simulink model "hcu_main_ADASwEPS"  (Simulink 8.2)
settings: Solver=FixedStepDiscrete  StartTime=0.0  StopTime=inf  FixedStep=0.001  RelTol=1e-3
PostLoadFcn:
  | , if any(exist('dsrtsu_mdlpostloadfcn', 'file') == [2, 3, 6]), try dsrtsu_mdlpostloadfcn('Execute', bdroot); catch fprintf('Error in PostLoadFcn (dsrtsu_mdlpostloadfcn) for model "%s":\n %s\n', bdroot, lasterr); end, end,
values from neighbouring files (symbols this model uses):
  C_TASK_1MS_S = (	C_TICK_TIME_S       )    [hcu_local_hdr.m]    (also in temp_ovrd_values.m = double(	0.001                  ))
  C_TICK_TIME_S = single(	0.005	    	)    [hcu_local_hdr.m]
  ENUM_EPSLFCSTATUS_ACTIVE = uint8(  2  )    [hcu_local_hdr.m]
  ENUM_EPSLFCSTATUS_TRANSITION = uint8(  3  )    [hcu_local_hdr.m]
  ENUM_EPSLKASTATUS_ACTIVE = uint8(  2  )    [hcu_local_hdr.m]
  ENUM_EPSMODEREQ_ANGLE = uint8(  1  )    [hcu_local_hdr.m]
  ENUM_EPSMODEREQ_INTERNAL = uint8(  0  )    [hcu_local_hdr.m]
  ENUM_EPSMODEREQ_TORQUE = uint8(  2  )    [hcu_local_hdr.m]
  ENUM_GEARPOSN_1ST = uint8(  1  )    [hcu_local_hdr.m]
  ENUM_GEARPOSN_2ND = uint8(  2  )    [hcu_local_hdr.m]
  ENUM_GEARPOSN_3RD = uint8(  3  )    [hcu_local_hdr.m]
  ENUM_GEARPOSN_4TH = uint8(  4  )    [hcu_local_hdr.m]
  ENUM_GEARPOSN_5TH = uint8(  5  )    [hcu_local_hdr.m]
  ENUM_GEARPOSN_6TH = uint8(  6  )    [hcu_local_hdr.m]
  ENUM_GEARPOSN_R = uint8(  7  )    [hcu_local_hdr.m]
  FALSE = boolean( 0 )    [hcu_local_hdr.m]
  TRUE = boolean( 1 )    [hcu_local_hdr.m]
undefined symbols (not defined in the file or in its folder): AISP_EPSCurrent_pct, AISP_TqASensorDelta_pct, AISP_TqBSensorDelta_pct, dHAL_IN, hal, INVALID_ABS1_TIMEOUT, INVALID_ABS2_TIMEOUT, INVALID_ABS3_TIMEOUT, INVALID_ABS4_TIMEOUT, INVALID_AC1_TIMEOUT, INVALID_ADASTORQ_REQ, INVALID_BCM1_TIMEOUT, INVALID_BCM2_TIMEOUT, INVALID_BOOSTER_VAC, INVALID_CSW1_TIMEOUT, INVALID_CUR_VEHDECE, INVALID_CURBRAKEDECE_REQ, INVALID_CURSTEERANG_REQ, INVALID_CURSTEERTQ_REQ, INVALID_ECM1_TIMEOUT, INVALID_ECM2_TIMEOUT, INVALID_ECM3_TIMEOUT, INVALID_ECM9_TIMEOUT, INVALID_ENG_TORQUE_FRICTIONAL, INVALID_ENG_TORQUE_INDICATED, INVALID_ENG_TORQUE_INDICATEDCOR, INVALID_ENG_TQ_MAX, INVALID_ENG_TQ_MIN, INVALID_EPAS2_TIMEOUT, INVALID_EPAS3_TIMEOUT, INVALID_EPB1_TIMEOUT, INVALID_EPS_BATTVOLT, INVALID_ESC_BATTVOLT, INVALID_GRADE, INVALID_HCU3_TIMEOUT, INVALID_HCU4_TIMEOUT, INVALID_HMI1_TIMEOUT, INVALID_HMI2_TIMEOUT, INVALID_LAT_ACC, INVALID_LONG_ACC, INVALID_MC_PRESSURE, INVALID_METER1_TIMEOUT, INVALID_METER3_TIMEOUT, INVALID_METER_VEHSPD, INVALID_ODO_METER, INVALID_OUTSIDE_TEMP, INVALID_PARKBRAKEBIND_STAT, INVALID_PEDALTQ_REQ, INVALID_SAS1_TIMEOUT, INVALID_SAS_ANGLE, INVALID_SHIFTER_POSN, INVALID_TCM1_TIMEOUT, INVALID_TCM2_TIMEOUT, INVALID_VCU1_TIMEOUT, INVALID_VCU2_TIMEOUT, INVALID_VEH_CRASH, INVALID_VEH_SPD, INVALID_WHEEL_SPD, INVALID_YAW_RATE, KHAL_MssgIdObj1_num ... (+8)
libraries: simulink x147, hcu_lib x38, rti1401lib_dio_type3 x4, rtimmsu_dsrtlib x3, app x1, rtiethernetudplib x1, rti1401lib_adc_type4 x1, rti1401lib_dac_type3 x1, inp x1, lidr x1, outp x1
(part 11 of 15)

== system hcu_main_ADASwEPS/EPSS/EPSS/LFCStatusArbitration ==
  VISP_EPSModeReq_enum : Inport
  VEPSS_LFCContStatusAng_enum : Inport  Port=2
  VEPSS_LFCContStatusTq_enum : Inport  Port=3
  VEPSS_EPSLKAAbReason_enum : Inport  Port=4
  VEPSS_EPSLFCAbReasonAng_enum : Inport  Port=5
  VEPSS_EPSLFCAbReasonTq_enum : Inport  Port=6
  Constant1 : Constant  Value=ENUM_EPSMODEREQ_INTERNAL
  Constant6 : Constant  Value=ENUM_EPSMODEREQ_ANGLE
  Relational Operator1 : RelationalOperator  Operator===  OutDataTypeStr=boolean
  Relational Operator3 : RelationalOperator  Operator===  OutDataTypeStr=boolean
  Switch1 : Switch  Criteria=u2 ~= 0
  Switch2 : Switch  Criteria=u2 ~= 0
  Switch3 : Switch  Criteria=u2 ~= 0
  VEPSS_LFCContStatus_enum : Outport
  VEPSS_EPSADASAbReason_enum : Outport  Port=2
  wires:
  VISP_EPSModeReq_enum/1 -> Relational Operator1/1, Relational Operator3/1
  Constant6/1 -> Relational Operator3/2
  Relational Operator3/1 -> Switch2/2, Switch1/2
  VEPSS_LFCContStatusAng_enum/1 -> Switch1/1
  VEPSS_LFCContStatusTq_enum/1 -> Switch1/3
  Switch1/1 -> VEPSS_LFCContStatus_enum/1
  VEPSS_EPSLFCAbReasonAng_enum/1 -> Switch2/1
  VEPSS_EPSLFCAbReasonTq_enum/1 -> Switch2/3
  Constant1/1 -> Relational Operator1/2
  Switch2/1 -> Switch3/3
  VEPSS_EPSLKAAbReason_enum/1 -> Switch3/1
  Switch3/1 -> VEPSS_EPSADASAbReason_enum/1
  Relational Operator1/1 -> Switch3/2

== system hcu_main_ADASwEPS/EPSS/EPSS/PWM Output Limit ==
  VEPSS_SteerPWM_pct : Inport
  VISP_StrAng_deg : Inport  Port=2
  VISP_StrAngValid_flg : Inport  Port=3
  Data Type Conversion : DataTypeConversion
  KEPSS_LockLimitationDefault_rat : Constant  SampleTime=-1
  KEPSS_MotorDutyMaxLim_pct : Constant  Value=100  SampleTime=-1
  KEPSS_MotorDutyMinLim_pct : Constant  Value=-100  SampleTime=-1
  Limit : hcu_lib/Limit  SystemSampleTime=-1
  MEPSS_LockLimitation_rat : Lookup  InputValues=[-600 -540 0 540 600]  Table=[0.5 1 1 1 0.5]  LookUpMeth=Interpolation-Use End Values
      settings: AttributesFormatString="Input=\"%<InputValues>\"\\nOutput=\"%<Table>\""
  Product : Product
  Switch : Switch  Criteria=u2 ~= 0
  VEPSS_MotorDuty_pct_over : hcu_lib/Signal_over  parent_name=VEPSS_MotorDuty_pct  cal=0
  VEPSS_MotorDuty_pct : Outport
  wires:
  VEPSS_SteerPWM_pct/1 -> Limit/1
  VEPSS_MotorDuty_pct_over/1 -> Data Type Conversion/1
  KEPSS_MotorDutyMaxLim_pct/1 -> Limit/2
  KEPSS_MotorDutyMinLim_pct/1 -> Limit/3
  Data Type Conversion/1 -> VEPSS_MotorDuty_pct/1  "VEPSS_MotorDuty_pct"
  VISP_StrAng_deg/1 -> MEPSS_LockLimitation_rat/1
  MEPSS_LockLimitation_rat/1 -> Switch/1
  VISP_StrAngValid_flg/1 -> Switch/2
  KEPSS_LockLimitationDefault_rat/1 -> Switch/3
  Limit/1 -> Product/1
  Product/1 -> VEPSS_MotorDuty_pct_over/1
  Switch/1 -> Product/2  "VEPSS_LockLimitation_rat"

== system hcu_main_ADASwEPS/EPSS/EPSS/ShaftTorqueProcessor ==
  VISP_EPSTqOnShaft_Nm : Inport
  AddLPF : Constant  Value=0
  Data Type Conversion : DataTypeConversion
  LowPassFilter_50ms : DiscreteTransferFcn  Numerator=[0 0.019801326693245]  Denominator=[1 -0.980198673306755]
  NotchFilter1 : DiscreteTransferFcn  Numerator=[1 -1.994058244407765 0.995032825431470]  Denominator=[1 -1.974205875760737 0.975180456784442]
  NotchFilter2 : DiscreteTransferFcn  Numerator=[1 -1.991175781675417 0.993076280925535]  Denominator=[1 -1.963525487771149 0.965425987021267]
  NotchFilter3 : DiscreteTransferFcn  Numerator=[1 -1.986359097364601 0.990196128638903]  Denominator=[1 -1.941183460066831 0.945020491341134]
  NotchFilter4 : DiscreteTransferFcn  Numerator=[1 -1.978872423909787 0.986339393241381]  Denominator=[1 -1.924580367084394 0.932047336415988]
  NotchFilter5 : DiscreteTransferFcn  Numerator=[1 -1.956033818662219 0.973851168649108]  Denominator=[1 -1.853080945250230 0.870898295237120]
  Switch : Switch  Criteria=u2 ~= 0
  VEPSS_EPSTqOnShaftRaw_Nm : Outport
  VEPSS_EPSTqOnShaftFlt_Nm : Outport  Port=2
  wires:
  VISP_EPSTqOnShaft_Nm/1 -> Data Type Conversion/1, NotchFilter1/1
  NotchFilter1/1 -> NotchFilter2/1
  NotchFilter2/1 -> NotchFilter3/1
  NotchFilter3/1 -> NotchFilter4/1
  NotchFilter4/1 -> NotchFilter5/1
  NotchFilter5/1 -> LowPassFilter_50ms/1, Switch/3
  Data Type Conversion/1 -> VEPSS_EPSTqOnShaftRaw_Nm/1  "VEPSS_EPSTqOnShaftRaw_Nm"
  Switch/1 -> VEPSS_EPSTqOnShaftFlt_Nm/1  "VEPSS_EPSTqOnShaftFlt_Nm"
  LowPassFilter_50ms/1 -> Switch/1
  AddLPF/1 -> Switch/2

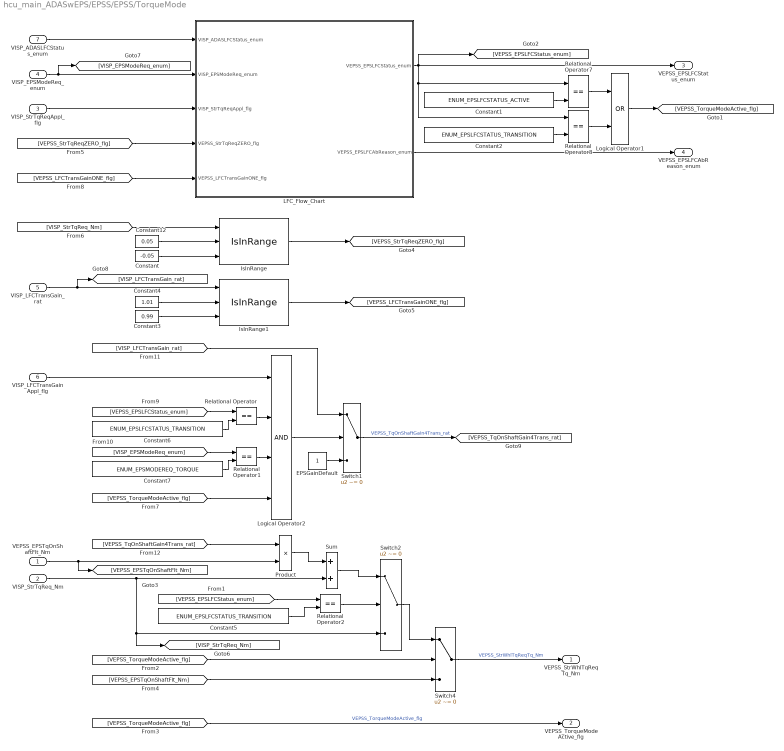
== system hcu_main_ADASwEPS/EPSS/EPSS/TorqueMode ==
  VEPSS_EPSTqOnShaftFlt_Nm : Inport
  VISP_StrTqReq_Nm : Inport  Port=2
  VISP_StrTqReqAppl_flg : Inport  Port=3
  VISP_EPSModeReq_enum : Inport  Port=4
  VISP_LFCTransGain_rat : Inport  Port=5
  VISP_LFCTransGainAppl_flg : Inport  Port=6
  VISP_ADASLFCStatus_enum : Inport  Port=7
  Constant : Constant  Value=-0.05
  Constant1 : Constant  Value=ENUM_EPSLFCSTATUS_ACTIVE
  Constant12 : Constant  Value=0.05
  Constant2 : Constant  Value=ENUM_EPSLFCSTATUS_TRANSITION
  Constant3 : Constant  Value=0.99
  Constant4 : Constant  Value=1.01
  Constant5 : Constant  Value=ENUM_EPSLFCSTATUS_TRANSITION
  Constant6 : Constant  Value=ENUM_EPSLFCSTATUS_TRANSITION
  Constant7 : Constant  Value=ENUM_EPSMODEREQ_TORQUE
  EPSGainDefault : Constant
  IsInRange : hcu_lib/IsInRange  SystemSampleTime=-1
  IsInRange1 : hcu_lib/IsInRange  SystemSampleTime=-1
  LFC_Flow_Chart : Stateflow chart  TreatAsAtomicUnit=on
  Logical Operator1 : Logic  Operator=OR  AllPortsSameDT=off  OutDataTypeStr=boolean
  Logical Operator2 : Logic  Inputs=4  AllPortsSameDT=off  OutDataTypeStr=boolean
  Product : Product
  Relational Operator{,1..2,7..8} (5 alike) : RelationalOperator  Operator===  OutDataTypeStr=boolean
  Sum : Sum
  Switch1 : Switch  Criteria=u2 ~= 0
  Switch2 : Switch  Criteria=u2 ~= 0
  Switch4 : Switch  Criteria=u2 ~= 0
  VEPSS_StrWhlTqReqTq_Nm : Outport
  VEPSS_TorqueModeActive_flg : Outport  Port=2
  VEPSS_EPSLFCStatus_enum : Outport  Port=3
  VEPSS_EPSLFCAbReason_enum : Outport  Port=4
  wires:
  Sum/1 -> Switch2/1
  VISP_StrTqReq_Nm/1 -> [VISP_StrTqReq_Nm], Switch2/3, Sum/2
  Switch4/1 -> VEPSS_StrWhlTqReqTq_Nm/1  "VEPSS_StrWhlTqReqTq_Nm"
  VEPSS_EPSTqOnShaftFlt_Nm/1 -> [VEPSS_EPSTqOnShaftFlt_Nm], Product/2
  Switch2/1 -> Switch4/1
  [VEPSS_TorqueModeActive_flg] -> Switch4/2
  [VEPSS_EPSLFCStatus_enum] -> Relational Operator2/1
  Constant5/1 -> Relational Operator2/2
  Relational Operator2/1 -> Switch2/2
  [VEPSS_EPSTqOnShaftFlt_Nm] -> Switch4/3
  [VEPSS_TorqueModeActive_flg] -> VEPSS_TorqueModeActive_flg/1  "VEPSS_TorqueModeActive_flg"
  [VISP_StrTqReq_Nm] -> IsInRange/1
  IsInRange/1 -> [VEPSS_StrTqReqZERO_flg]
  Constant/1 -> IsInRange/3
  Constant12/1 -> IsInRange/2
  LFC_Flow_Chart/1(VEPSS_EPSLFCStatus_enum) -> [VEPSS_EPSLFCStatus_enum], VEPSS_EPSLFCStatus_enum/1, Relational Operator8/1, Relational Operator7/1
  Constant1/1 -> Relational Operator7/2
  Constant2/1 -> Relational Operator8/2
  LFC_Flow_Chart/2(VEPSS_EPSLFCAbReason_enum) -> VEPSS_EPSLFCAbReason_enum/1
  Relational Operator8/1 -> Logical Operator1/2
  Relational Operator7/1 -> Logical Operator1/1
  Logical Operator1/1 -> [VEPSS_TorqueModeActive_flg]
  VISP_ADASLFCStatus_enum/1 -> LFC_Flow_Chart/1(VISP_ADASLFCStatus_enum)
  VISP_EPSModeReq_enum/1 -> [VISP_EPSModeReq_enum], LFC_Flow_Chart/2(VISP_EPSModeReq_enum)
  VISP_StrTqReqAppl_flg/1 -> LFC_Flow_Chart/3(VISP_StrTqReqAppl_flg)
  [VEPSS_StrTqReqZERO_flg] -> LFC_Flow_Chart/4(VEPSS_StrTqReqZERO_flg)
  VISP_LFCTransGain_rat/1 -> [VISP_LFCTransGain_rat], IsInRange1/1
  IsInRange1/1 -> [VEPSS_LFCTransGainONE_flg]
  Constant3/1 -> IsInRange1/3
  Constant4/1 -> IsInRange1/2
  [VEPSS_LFCTransGainONE_flg] -> LFC_Flow_Chart/5(VEPSS_LFCTransGainONE_flg)
  [VEPSS_EPSLFCStatus_enum] -> Relational Operator/1
  Constant6/1 -> Relational Operator/2
  VISP_LFCTransGainAppl_flg/1 -> Logical Operator2/1
  Relational Operator/1 -> Logical Operator2/2
  [VEPSS_TorqueModeActive_flg] -> Logical Operator2/4
  Logical Operator2/1 -> Switch1/2
  Switch1/1 -> [VEPSS_TqOnShaftGain4Trans_rat]  "VEPSS_TqOnShaftGain4Trans_rat"
  EPSGainDefault/1 -> Switch1/3
  [VISP_EPSModeReq_enum] -> Relational Operator1/1
  Constant7/1 -> Relational Operator1/2
  Relational Operator1/1 -> Logical Operator2/3
  [VISP_LFCTransGain_rat] -> Switch1/1
  Product/1 -> Sum/1
  [VEPSS_TqOnShaftGain4Trans_rat] -> Product/1

== system hcu_main_ADASwEPS/EPSS/model_info/EmptySubsystem ==

== system hcu_main_ADASwEPS/ISP/AngleProcessing/Timer ==
  Enable : EnablePort  StatesWhenEnabling=reset
  C_TASK_1MS_S : Constant  Value=C_TASK_1MS_S
  Sum : Sum  Inputs=|++
  Unit Delay : UnitDelay  SampleTime=-1
  Unit Delay1 : UnitDelay  SampleTime=-1
  Time_s : Outport  OutputWhenDisabled=reset  InitialOutput=[0]
  wires:
  C_TASK_1MS_S/1 -> Unit Delay1/1
  Sum/1 -> Unit Delay/1, Time_s/1  "Time_s"
  Unit Delay/1 -> Sum/2
  Unit Delay1/1 -> Sum/1

== system hcu_main_ADASwEPS/ISP/AngleProcessing/Triggered Absolute Angle Zero ==
  In : Inport
  Trigger : TriggerPort
  SteerAngValid_flg : Constant  Value=TRUE
  Out1 : Outport
  Out2 : Outport  Port=2
  wires:
  In/1 -> Out1/1
  SteerAngValid_flg/1 -> Out2/1

== system hcu_main_ADASwEPS/ISP/PassThrough/EPSDegTest ==
  PassThrough : Inport
  AmplitudeDeg_pct : Constant  Value=5
  Compare To Constant : simulink/Logic and Bit Operations/Compare To Constant  relop===  const=3.0  OutDataTypeStr=boolean
  Constant : Constant  Value=2*pi  OutDataTypeStr=single
  DegSetPt : Constant
  FrequencyDeg_Hz : Constant
  Multiport Switch1 : MultiPortSwitch  Inputs=4
  Product : Product  Inputs=3  RndMeth=Zero
  Product1 : Product  RndMeth=Zero
  TestModeDeg_Sw : Constant
  Timer : Subsystem
  Trigonometric Funcon : Trigonometry
  DegOut : Outport
  wires:
  Multiport Switch1/1 -> DegOut/1  "DegOut"
  PassThrough/1 -> Multiport Switch1/2
  DegSetPt/1 -> Multiport Switch1/3
  Product1/1 -> Multiport Switch1/4
  FrequencyDeg_Hz/1 -> Product/2
  Product/1 -> Trigonometric Funcon/1
  AmplitudeDeg_pct/1 -> Product1/2
  Trigonometric Funcon/1 -> Product1/1
  Constant/1 -> Product/3
  Timer/1(SineTime_s) -> Product/1
  TestModeDeg_Sw/1 -> Compare To Constant/1, Multiport Switch1/1
  Compare To Constant/1 -> Timer/Enable

== system hcu_main_ADASwEPS/ISP/TqProcessing/LowPassFilter ==
  Raw : Inport
  Constant1 : Constant  OutDataTypeStr=single  SampleTime=-1
  LowPassCoef : Constant  SampleTime=-1
  Product : Product  RndMeth=Zero
  Product1 : Product  RndMeth=Zero
  Sum1 : Sum  Inputs=+-
  Sum2 : Sum
  Unit Delay1 : UnitDelay  SampleTime=-1
  Out : Outport
  wires:
  Raw/1 -> Product/2
  Constant1/1 -> Sum1/1
  LowPassCoef/1 -> [LowPassCoef], Product/1
  [LowPassCoef] -> Sum1/2
  Unit Delay1/1 -> Product1/1
  Sum1/1 -> Product1/2
  Product/1 -> Sum2/1
  Product1/1 -> Sum2/2
  Sum2/1 -> Unit Delay1/1, Out/1

== system hcu_main_ADASwEPS/ISP/TqProcessing/TorqueValid ==
  TqA : Inport
  TqB : Inport  Port=2
  Abs1 : Abs
  FALSE : Constant  Value=FALSE  OutDataTypeStr=single  SampleTime=-1
  Relational Operator1 : RelationalOperator  Operator=<=  OutDataTypeStr=boolean
  Sum1 : Sum  Inputs=+-
  Switch1 : Switch  Criteria=u2 ~= 0
  TRUE : Constant  Value=TRUE  OutDataTypeStr=single  SampleTime=-1
  TqValidThres_Nm : Constant  OutDataTypeStr=single  SampleTime=-1
  TqValid_flg : Outport
  wires:
  TRUE/1 -> Switch1/1
  TqValidThres_Nm/1 -> Relational Operator1/2
  Relational Operator1/1 -> Switch1/2
  Sum1/1 -> Abs1/1
  Abs1/1 -> Relational Operator1/1
  FALSE/1 -> Switch1/3
  Switch1/1 -> TqValid_flg/1  "TqValid_flg"
  TqA/1 -> Sum1/1
  TqB/1 -> Sum1/2

== system hcu_main_ADASwEPS/ISP/TqProcessing/TqSensorAZero ==
  VHAL_TqSensorADuty_pct : Inport
  TqSensorFlac_pct : Inport  Port=2
  KISP_EPSZeroReset_flg : Inport  Port=3
  Constant1 : Constant  Value=60  OutDataTypeStr=single  SampleTime=-1
  Constant2 : Constant  Value=50  OutDataTypeStr=single  SampleTime=-1
  Delay : Delay  DelayLength=1  InitialCondition=0
  Delay1 : Delay  DelayLength=1  InitialCondition=1
  Delay2 : Delay  DelayLength=1  InitialCondition=1
  FALSE : Constant  Value=FALSE
  Gain : Gain  Gain=-1
  IsInRange : hcu_lib/IsInRange  SystemSampleTime=-1
  IsInRange1 : hcu_lib/IsInRange  SystemSampleTime=-1
  KISP_CheckZeroTime_s : Constant  Value=3
  Latch : Subsystem
  Logical Operator : Logic  Operator=NOT  AllPortsSameDT=off  OutDataTypeStr=boolean
  Logical Operator1 : Logic  Operator=OR  AllPortsSameDT=off  OutDataTypeStr=boolean
  Logical Operator4 : Logic  AllPortsSameDT=off  OutDataTypeStr=boolean
  Relational Operator : RelationalOperator  Operator=<=  OutDataTypeStr=boolean
  Subtract : Sum  Inputs=+-
  Subtract1 : Sum  Inputs=+-
  Switch : Switch  Criteria=u2 ~= 0
  Switch1 : Switch  Criteria=u2 ~= 0
  Timer : Subsystem
  zero : Outport
  delta : Outport  Port=2
  wires:
  Relational Operator/1 -> Switch/2
  Logical Operator1/1 -> Latch/2(update)
  KISP_EPSZeroReset_flg/1 -> Logical Operator1/1
  Delay1/1 -> Logical Operator1/2
  Latch/1(out) -> Subtract/2, Switch/3
  Switch/1 -> Delay/1, Subtract1/2, zero/1
  KISP_CheckZeroTime_s/1 -> Relational Operator/2
  Timer/1(Time_s) -> Relational Operator/1
  Subtract/1 -> IsInRange/1
  VHAL_TqSensorADuty_pct/1 -> Subtract/1, IsInRange1/1, Switch1/1, Subtract1/1, Latch/1(in)
  Gain/1 -> IsInRange/3
  TqSensorFlac_pct/1 -> IsInRange/2, Gain/1
  Subtract1/1 -> delta/1
  IsInRange/1 -> Logical Operator4/2, Logical Operator/1
  Switch1/1 -> Switch/1
  Logical Operator/1 -> Delay1/1
  FALSE/1 -> Delay2/1
  Delay2/1 -> Switch1/2
  Delay/1 -> Switch1/3
  Logical Operator4/1 -> Timer/Enable
  IsInRange1/1 -> Logical Operator4/1
  Constant1/1 -> IsInRange1/2
  Constant2/1 -> IsInRange1/3

== system hcu_main_ADASwEPS/ISP/TqProcessing/TqSensorBZero ==
  VHAL_TqSensorBDuty_pct : Inport
  TqSensorFlac_pct : Inport  Port=2
  KISP_EPSZeroReset_flg : Inport  Port=3
  Constant1 : Constant  Value=60  OutDataTypeStr=single  SampleTime=-1
  Constant2 : Constant  Value=50  OutDataTypeStr=single  SampleTime=-1
  Delay : Delay  DelayLength=1  InitialCondition=0
  Delay1 : Delay  DelayLength=1  InitialCondition=1
  Delay2 : Delay  DelayLength=1  InitialCondition=1
  FALSE : Constant  Value=FALSE
  Gain : Gain  Gain=-1
  IsInRange : hcu_lib/IsInRange  SystemSampleTime=-1
  IsInRange1 : hcu_lib/IsInRange  SystemSampleTime=-1
  KISP_CheckZeroTime_s : Constant  Value=3
  Latch : Subsystem
  Logical Operator : Logic  Operator=NOT  AllPortsSameDT=off  OutDataTypeStr=boolean
  Logical Operator1 : Logic  Operator=OR  AllPortsSameDT=off  OutDataTypeStr=boolean
  Logical Operator4 : Logic  AllPortsSameDT=off  OutDataTypeStr=boolean
  Relational Operator : RelationalOperator  Operator=<=  OutDataTypeStr=boolean
  Subtract : Sum  Inputs=+-
  Subtract1 : Sum  Inputs=+-
  Switch : Switch  Criteria=u2 ~= 0
  Switch1 : Switch  Criteria=u2 ~= 0
  Timer : Subsystem
  zero : Outport
  delta : Outport  Port=2
  wires:
  Constant2/1 -> IsInRange1/3
  Constant1/1 -> IsInRange1/2
  IsInRange1/1 -> Logical Operator4/1
  Logical Operator4/1 -> Timer/Enable
  Delay/1 -> Switch1/3
  Delay2/1 -> Switch1/2
  FALSE/1 -> Delay2/1
  Logical Operator/1 -> Delay1/1
  Switch1/1 -> Switch/1
  IsInRange/1 -> Logical Operator/1, Logical Operator4/2
  Subtract1/1 -> delta/1
  TqSensorFlac_pct/1 -> IsInRange/2, Gain/1
  Gain/1 -> IsInRange/3
  VHAL_TqSensorBDuty_pct/1 -> Subtract/1, IsInRange1/1, Subtract1/1, Switch1/1, Latch/1(in)
  Subtract/1 -> IsInRange/1
  Timer/1(Time_s) -> Relational Operator/1
  KISP_CheckZeroTime_s/1 -> Relational Operator/2
  Switch/1 -> zero/1, Subtract1/2, Delay/1
  Latch/1(out) -> Switch/3, Subtract/2
  Delay1/1 -> Logical Operator1/2
  KISP_EPSZeroReset_flg/1 -> Logical Operator1/1
  Logical Operator1/1 -> Latch/2(update)
  Relational Operator/1 -> Switch/2

== system hcu_main_ADASwEPS/OSP/OSP/CheckSum Calculation ==
  BISP_outputs : Inport
  LifeCount : Inport  Port=2
  Byte0 : Subsystem
  Byte1 : Subsystem
  Byte2 : Subsystem
  Byte3 : Subsystem
  ChecksumCalculation : Subsystem  TreatAsAtomicUnit=on
  VOSP_SAS1CalcChecksum_raw8 : Outport
  wires:
  Byte0/2(ForByte1) -> Byte1/1(ForByte1)
  BISP_outputs/1 -> Byte0/1(BISP_outputs), Byte3/1(BISP_outputs)
  LifeCount/1 -> ChecksumCalculation/5(SAS_MsgCount)
  ChecksumCalculation/1(Message_Checksum) -> VOSP_SAS1CalcChecksum_raw8/1  "VOSP_SAS1CalcChecksum_raw8"
  Byte0/1(Byte0) -> ChecksumCalculation/1(Byte0)
  Byte1/1(Byte1) -> ChecksumCalculation/2(Byte1)
  Byte3/1(Byte3) -> ChecksumCalculation/4(Byte3)
  Byte2/1(Byte2) -> ChecksumCalculation/3(Byte2)

== system hcu_main_ADASwEPS/OSP/OSP/CheckSum Calculation1 ==
  BEPSS_outputs : Inport
  BISP_outputs : Inport  Port=2
  LifeCount : Inport  Port=3
  Byte0 : Subsystem
  Byte1 : Subsystem
  Byte2 : Subsystem
  Byte3 : Subsystem
  ChecksumCalculation : Subsystem  TreatAsAtomicUnit=on
  VOSP_EPAS2CalcChecksum_raw8 : Outport
  wires:
  ChecksumCalculation/1(Message_Checksum) -> VOSP_EPAS2CalcChecksum_raw8/1  "VOSP_EPAS2CalcChecksum_raw8"
  LifeCount/1 -> ChecksumCalculation/6(EPAS2_MsgCount)
  BISP_outputs/1 -> Byte3/1(BISP_outputs), Byte1/1(BISP_outputs)
  Byte0/1(Byte0) -> ChecksumCalculation/1(Byte0)
  Byte1/1(Byte1) -> ChecksumCalculation/2(Byte1)
  Byte2/1(Byte2) -> ChecksumCalculation/3(Byte2)
  Byte3/1(Byte3) -> ChecksumCalculation/4(Byte3)
  Byte3/2(ForByte4) -> ChecksumCalculation/5(Byte4)
  BEPSS_outputs/1 -> Byte2/1(BEPSS_outputs)

== system hcu_main_ADASwEPS/OSP/OSP/CheckSum Calculation2 ==
  BEPSS_outputs : Inport
  LifeCount : Inport  Port=2
  Byte0 : Subsystem
  Byte1 : Subsystem
  Byte2 : Subsystem
  Byte3 : Subsystem
  Byte4 : Subsystem
  Byte5 : Subsystem
  Byte6 : Subsystem
  ChecksumCalculation : Subsystem  TreatAsAtomicUnit=on
  VOSP_EPAS3CalcChecksum_raw8 : Outport
  wires:
  Byte2/1(Byte2) -> ChecksumCalculation/3(Byte2)
  Byte3/1(Byte3) -> ChecksumCalculation/4(Byte3)
  Byte1/1(Byte1) -> ChecksumCalculation/2(Byte1)
  Byte0/1(Byte0) -> ChecksumCalculation/1(Byte0)
  ChecksumCalculation/1(Message_Checksum) -> VOSP_EPAS3CalcChecksum_raw8/1  "VOSP_EPAS3CalcChecksum_raw8"
  LifeCount/1 -> ChecksumCalculation/8(SAS_MsgCount)
  BEPSS_outputs/1 -> Byte2/1(BEPSS_outputs), Byte6/1(BEPSS_outputs), Byte4/1(BEPSS_outputs), Byte0/1(BEPSS_outputs)
  Byte0/2(ForByte1) -> Byte1/1(ForByte1)
  Byte4/1(Byte4) -> ChecksumCalculation/5(Byte4)
  Byte5/1(Byte5) -> ChecksumCalculation/6(Byte5)
  Byte6/1(Byte6) -> ChecksumCalculation/7(Byte6)

== system hcu_main_ADASwEPS/OSP/OSP/RollCnt ==
  max : Inport
  Trigger : TriggerPort  TriggerType=function-call  PortDimensions=1
  Add : Sum
  Constant : Constant  OutDataTypeStr=Inherit: Inherit via back propagation
  Constant1 : Constant  Value=0  OutDataTypeStr=Inherit: Inherit via back propagation
  Data Type Conversion6 : DataTypeConversion  OutDataTypeStr=uint8
  Relational Operator : RelationalOperator  Operator=>  OutDataTypeStr=boolean
  Switch2 : Switch  Criteria=u2 ~= 0
  Unit Delay1 : UnitDelay  SampleTime=-1
  out : Outport
  wires:
  Constant/1 -> Add/1
  Add/1 -> Switch2/3, Relational Operator/1
  Unit Delay1/1 -> Add/2
  Constant1/1 -> Switch2/1
  Switch2/1 -> Unit Delay1/1, Data Type Conversion6/1
  max/1 -> Relational Operator/2
  Relational Operator/1 -> Switch2/2
  Data Type Conversion6/1 -> out/1

== system hcu_main_ADASwEPS/OSP/OSP/RollCnt1 ==
  max : Inport
  Trigger : TriggerPort  TriggerType=function-call  PortDimensions=1
  Add : Sum
  Constant : Constant  OutDataTypeStr=Inherit: Inherit via back propagation
  Constant1 : Constant  Value=0  OutDataTypeStr=Inherit: Inherit via back propagation
  Data Type Conversion6 : DataTypeConversion  OutDataTypeStr=uint8
  Relational Operator : RelationalOperator  Operator=>  OutDataTypeStr=boolean
  Switch2 : Switch  Criteria=u2 ~= 0
  Unit Delay1 : UnitDelay  SampleTime=-1
  out : Outport
  wires:
  Data Type Conversion6/1 -> out/1
  Relational Operator/1 -> Switch2/2
  max/1 -> Relational Operator/2
  Switch2/1 -> Data Type Conversion6/1, Unit Delay1/1
  Constant1/1 -> Switch2/1
  Unit Delay1/1 -> Add/2
  Add/1 -> Relational Operator/1, Switch2/3
  Constant/1 -> Add/1

== system hcu_main_ADASwEPS/OSP/OSP/RollCnt2 ==
  max : Inport
  Trigger : TriggerPort  TriggerType=function-call  PortDimensions=1
  Add : Sum
  Constant : Constant  OutDataTypeStr=Inherit: Inherit via back propagation
  Constant1 : Constant  Value=0  OutDataTypeStr=Inherit: Inherit via back propagation
  Data Type Conversion6 : DataTypeConversion  OutDataTypeStr=uint8
  Relational Operator : RelationalOperator  Operator=>  OutDataTypeStr=boolean
  Switch2 : Switch  Criteria=u2 ~= 0
  Unit Delay1 : UnitDelay  SampleTime=-1
  out : Outport
  wires:
  Constant/1 -> Add/1
  Add/1 -> Switch2/3, Relational Operator/1
  Unit Delay1/1 -> Add/2
  Constant1/1 -> Switch2/1
  Switch2/1 -> Unit Delay1/1, Data Type Conversion6/1
  max/1 -> Relational Operator/2
  Relational Operator/1 -> Switch2/2
  Data Type Conversion6/1 -> out/1

== system hcu_main_ADASwEPS/RTI Data/RTI Data Store/RTI Data Store ==
  RTI Data Store : Subsystem  mask(RTI_DATA_STORE){}
      mask help:
      | RTI Data Store Block. This block is used by RTI to store internal model dependent data. Deleting this block will result in data loss.
      |
      | NEVER DELETE, COPY, OR MODIFY THIS BLOCK!
      mask Help:
      | RTI Data Store Block. This block is used by RTI to store internal model dependent data. Deleting this block will result in data loss.
      | 
      | NEVER DELETE, COPY, OR MODIFY THIS BLOCK!
      mask Display: text(0.5, 0.5, ' ', 'HorizontalAlignment', 'center');

== system hcu_main_ADASwEPS/dHAL_IN/HAL_IN_CANVALID/ChaekCANValid ==
  Rx_status : Inport
  TimeOut : Inport  Port=2
  Logical Operator : Logic  Operator=NOT  AllPortsSameDT=off  OutDataTypeStr=boolean
  Relational Operator : RelationalOperator  Operator=<=  OutDataTypeStr=boolean
  Timer : hcu_lib/Timer  SystemSampleTime=-1
  Valid_out : Outport
  wires:
  Timer/1 -> Relational Operator/1
  Rx_status/1 -> Logical Operator/1
  Logical Operator/1 -> Timer/Enable
  Relational Operator/1 -> Valid_out/1
  TimeOut/1 -> Relational Operator/2

== system hcu_main_ADASwEPS/dHAL_IN/HAL_IN_CANVALID/ChaekCANValid1 ==
  Rx_status : Inport
  TimeOut : Inport  Port=2
  Logical Operator : Logic  Operator=NOT  AllPortsSameDT=off  OutDataTypeStr=boolean
  Relational Operator : RelationalOperator  Operator=<=  OutDataTypeStr=boolean
  Timer : hcu_lib/Timer  SystemSampleTime=-1
  Valid_out : Outport
  wires:
  TimeOut/1 -> Relational Operator/2
  Relational Operator/1 -> Valid_out/1
  Logical Operator/1 -> Timer/Enable
  Rx_status/1 -> Logical Operator/1
  Timer/1 -> Relational Operator/1

== system hcu_main_ADASwEPS/dHAL_IN/HAL_IN_CANVALID/ChaekCANValid10 ==
  Rx_status : Inport
  TimeOut : Inport  Port=2
  Logical Operator : Logic  Operator=NOT  AllPortsSameDT=off  OutDataTypeStr=boolean
  Relational Operator : RelationalOperator  Operator=<=  OutDataTypeStr=boolean
  Timer : hcu_lib/Timer  SystemSampleTime=-1
  Valid_out : Outport
  wires:
  TimeOut/1 -> Relational Operator/2
  Relational Operator/1 -> Valid_out/1
  Logical Operator/1 -> Timer/Enable
  Rx_status/1 -> Logical Operator/1
  Timer/1 -> Relational Operator/1

== system hcu_main_ADASwEPS/dHAL_IN/HAL_IN_CANVALID/ChaekCANValid11 ==
  Rx_status : Inport
  TimeOut : Inport  Port=2
  Logical Operator : Logic  Operator=NOT  AllPortsSameDT=off  OutDataTypeStr=boolean
  Relational Operator : RelationalOperator  Operator=<=  OutDataTypeStr=boolean
  Timer : hcu_lib/Timer  SystemSampleTime=-1
  Valid_out : Outport
  wires:
  Timer/1 -> Relational Operator/1
  Rx_status/1 -> Logical Operator/1
  Logical Operator/1 -> Timer/Enable
  Relational Operator/1 -> Valid_out/1
  TimeOut/1 -> Relational Operator/2

== system hcu_main_ADASwEPS/dHAL_IN/HAL_IN_CANVALID/ChaekCANValid12 ==
  Rx_status : Inport
  TimeOut : Inport  Port=2
  Logical Operator : Logic  Operator=NOT  AllPortsSameDT=off  OutDataTypeStr=boolean
  Relational Operator : RelationalOperator  Operator=<=  OutDataTypeStr=boolean
  Timer : hcu_lib/Timer  SystemSampleTime=-1
  Valid_out : Outport
  wires:
  TimeOut/1 -> Relational Operator/2
  Relational Operator/1 -> Valid_out/1
  Logical Operator/1 -> Timer/Enable
  Rx_status/1 -> Logical Operator/1
  Timer/1 -> Relational Operator/1

== system hcu_main_ADASwEPS/dHAL_IN/HAL_IN_CANVALID/ChaekCANValid13 ==
  Rx_status : Inport
  TimeOut : Inport  Port=2
  Logical Operator : Logic  Operator=NOT  AllPortsSameDT=off  OutDataTypeStr=boolean
  Relational Operator : RelationalOperator  Operator=<=  OutDataTypeStr=boolean
  Timer : hcu_lib/Timer  SystemSampleTime=-1
  Valid_out : Outport
  wires:
  Timer/1 -> Relational Operator/1
  Rx_status/1 -> Logical Operator/1
  Logical Operator/1 -> Timer/Enable
  Relational Operator/1 -> Valid_out/1
  TimeOut/1 -> Relational Operator/2

== system hcu_main_ADASwEPS/dHAL_IN/HAL_IN_CANVALID/ChaekCANValid14 ==
  Rx_status : Inport
  TimeOut : Inport  Port=2
  Logical Operator : Logic  Operator=NOT  AllPortsSameDT=off  OutDataTypeStr=boolean
  Relational Operator : RelationalOperator  Operator=<=  OutDataTypeStr=boolean
  Timer : hcu_lib/Timer  SystemSampleTime=-1
  Valid_out : Outport
  wires:
  Timer/1 -> Relational Operator/1
  Rx_status/1 -> Logical Operator/1
  Logical Operator/1 -> Timer/Enable
  Relational Operator/1 -> Valid_out/1
  TimeOut/1 -> Relational Operator/2

== system hcu_main_ADASwEPS/dHAL_IN/HAL_IN_CANVALID/ChaekCANValid15 ==
  Rx_status : Inport
  TimeOut : Inport  Port=2
  Logical Operator : Logic  Operator=NOT  AllPortsSameDT=off  OutDataTypeStr=boolean
  Relational Operator : RelationalOperator  Operator=<=  OutDataTypeStr=boolean
  Timer : hcu_lib/Timer  SystemSampleTime=-1
  Valid_out : Outport
  wires:
  TimeOut/1 -> Relational Operator/2
  Relational Operator/1 -> Valid_out/1
  Logical Operator/1 -> Timer/Enable
  Rx_status/1 -> Logical Operator/1
  Timer/1 -> Relational Operator/1

== system hcu_main_ADASwEPS/dHAL_IN/HAL_IN_CANVALID/ChaekCANValid16 ==
  Rx_status : Inport
  TimeOut : Inport  Port=2
  Logical Operator : Logic  Operator=NOT  AllPortsSameDT=off  OutDataTypeStr=boolean
  Relational Operator : RelationalOperator  Operator=<=  OutDataTypeStr=boolean
  Timer : hcu_lib/Timer  SystemSampleTime=-1
  Valid_out : Outport
  wires:
  Timer/1 -> Relational Operator/1
  Rx_status/1 -> Logical Operator/1
  Logical Operator/1 -> Timer/Enable
  Relational Operator/1 -> Valid_out/1
  TimeOut/1 -> Relational Operator/2

== system hcu_main_ADASwEPS/dHAL_IN/HAL_IN_CANVALID/ChaekCANValid17 ==
  Rx_status : Inport
  TimeOut : Inport  Port=2
  Logical Operator : Logic  Operator=NOT  AllPortsSameDT=off  OutDataTypeStr=boolean
  Relational Operator : RelationalOperator  Operator=<=  OutDataTypeStr=boolean
  Timer : hcu_lib/Timer  SystemSampleTime=-1
  Valid_out : Outport
  wires:
  Timer/1 -> Relational Operator/1
  Rx_status/1 -> Logical Operator/1
  Logical Operator/1 -> Timer/Enable
  Relational Operator/1 -> Valid_out/1
  TimeOut/1 -> Relational Operator/2

== system hcu_main_ADASwEPS/dHAL_IN/HAL_IN_CANVALID/ChaekCANValid18 ==
  Rx_status : Inport
  TimeOut : Inport  Port=2
  Logical Operator : Logic  Operator=NOT  AllPortsSameDT=off  OutDataTypeStr=boolean
  Relational Operator : RelationalOperator  Operator=<=  OutDataTypeStr=boolean
  Timer : hcu_lib/Timer  SystemSampleTime=-1
  Valid_out : Outport
  wires:
  TimeOut/1 -> Relational Operator/2
  Relational Operator/1 -> Valid_out/1
  Logical Operator/1 -> Timer/Enable
  Rx_status/1 -> Logical Operator/1
  Timer/1 -> Relational Operator/1

== system hcu_main_ADASwEPS/dHAL_IN/HAL_IN_CANVALID/ChaekCANValid19 ==
  Rx_status : Inport
  TimeOut : Inport  Port=2
  Logical Operator : Logic  Operator=NOT  AllPortsSameDT=off  OutDataTypeStr=boolean
  Relational Operator : RelationalOperator  Operator=<=  OutDataTypeStr=boolean
  Timer : hcu_lib/Timer  SystemSampleTime=-1
  Valid_out : Outport
  wires:
  Timer/1 -> Relational Operator/1
  Rx_status/1 -> Logical Operator/1
  Logical Operator/1 -> Timer/Enable
  Relational Operator/1 -> Valid_out/1
  TimeOut/1 -> Relational Operator/2

== system hcu_main_ADASwEPS/dHAL_IN/HAL_IN_CANVALID/ChaekCANValid2 ==
  Rx_status : Inport
  TimeOut : Inport  Port=2
  Logical Operator : Logic  Operator=NOT  AllPortsSameDT=off  OutDataTypeStr=boolean
  Relational Operator : RelationalOperator  Operator=<=  OutDataTypeStr=boolean
  Timer : hcu_lib/Timer  SystemSampleTime=-1
  Valid_out : Outport
  wires:
  Timer/1 -> Relational Operator/1
  Rx_status/1 -> Logical Operator/1
  Logical Operator/1 -> Timer/Enable
  Relational Operator/1 -> Valid_out/1
  TimeOut/1 -> Relational Operator/2

== system hcu_main_ADASwEPS/dHAL_IN/HAL_IN_CANVALID/ChaekCANValid20 ==
  Rx_status : Inport
  TimeOut : Inport  Port=2
  Logical Operator : Logic  Operator=NOT  AllPortsSameDT=off  OutDataTypeStr=boolean
  Relational Operator : RelationalOperator  Operator=<=  OutDataTypeStr=boolean
  Timer : hcu_lib/Timer  SystemSampleTime=-1
  Valid_out : Outport
  wires:
  TimeOut/1 -> Relational Operator/2
  Relational Operator/1 -> Valid_out/1
  Logical Operator/1 -> Timer/Enable
  Rx_status/1 -> Logical Operator/1
  Timer/1 -> Relational Operator/1

== system hcu_main_ADASwEPS/dHAL_IN/HAL_IN_CANVALID/ChaekCANValid21 ==
  Rx_status : Inport
  TimeOut : Inport  Port=2
  Logical Operator : Logic  Operator=NOT  AllPortsSameDT=off  OutDataTypeStr=boolean
  Relational Operator : RelationalOperator  Operator=<=  OutDataTypeStr=boolean
  Timer : hcu_lib/Timer  SystemSampleTime=-1
  Valid_out : Outport
  wires:
  TimeOut/1 -> Relational Operator/2
  Relational Operator/1 -> Valid_out/1
  Logical Operator/1 -> Timer/Enable
  Rx_status/1 -> Logical Operator/1
  Timer/1 -> Relational Operator/1

== system hcu_main_ADASwEPS/dHAL_IN/HAL_IN_CANVALID/ChaekCANValid22 ==
  Rx_status : Inport
  TimeOut : Inport  Port=2
  Logical Operator : Logic  Operator=NOT  AllPortsSameDT=off  OutDataTypeStr=boolean
  Relational Operator : RelationalOperator  Operator=<=  OutDataTypeStr=boolean
  Timer : hcu_lib/Timer  SystemSampleTime=-1
  Valid_out : Outport
  wires:
  Timer/1 -> Relational Operator/1
  Rx_status/1 -> Logical Operator/1
  Logical Operator/1 -> Timer/Enable
  Relational Operator/1 -> Valid_out/1
  TimeOut/1 -> Relational Operator/2

== system hcu_main_ADASwEPS/dHAL_IN/HAL_IN_CANVALID/ChaekCANValid23 ==
  Rx_status : Inport
  TimeOut : Inport  Port=2
  Logical Operator : Logic  Operator=NOT  AllPortsSameDT=off  OutDataTypeStr=boolean
  Relational Operator : RelationalOperator  Operator=<=  OutDataTypeStr=boolean
  Timer : hcu_lib/Timer  SystemSampleTime=-1
  Valid_out : Outport
  wires:
  TimeOut/1 -> Relational Operator/2
  Relational Operator/1 -> Valid_out/1
  Logical Operator/1 -> Timer/Enable
  Rx_status/1 -> Logical Operator/1
  Timer/1 -> Relational Operator/1

== system hcu_main_ADASwEPS/dHAL_IN/HAL_IN_CANVALID/ChaekCANValid24 ==
  Rx_status : Inport
  TimeOut : Inport  Port=2
  Logical Operator : Logic  Operator=NOT  AllPortsSameDT=off  OutDataTypeStr=boolean
  Relational Operator : RelationalOperator  Operator=<=  OutDataTypeStr=boolean
  Timer : hcu_lib/Timer  SystemSampleTime=-1
  Valid_out : Outport
  wires:
  TimeOut/1 -> Relational Operator/2
  Relational Operator/1 -> Valid_out/1
  Logical Operator/1 -> Timer/Enable
  Rx_status/1 -> Logical Operator/1
  Timer/1 -> Relational Operator/1

== system hcu_main_ADASwEPS/dHAL_IN/HAL_IN_CANVALID/ChaekCANValid25 ==
  Rx_status : Inport
  TimeOut : Inport  Port=2
  Logical Operator : Logic  Operator=NOT  AllPortsSameDT=off  OutDataTypeStr=boolean
  Relational Operator : RelationalOperator  Operator=<=  OutDataTypeStr=boolean
  Timer : hcu_lib/Timer  SystemSampleTime=-1
  Valid_out : Outport
  wires:
  TimeOut/1 -> Relational Operator/2
  Relational Operator/1 -> Valid_out/1
  Logical Operator/1 -> Timer/Enable
  Rx_status/1 -> Logical Operator/1
  Timer/1 -> Relational Operator/1

== system hcu_main_ADASwEPS/dHAL_IN/HAL_IN_CANVALID/ChaekCANValid3 ==
  Rx_status : Inport
  TimeOut : Inport  Port=2
  Logical Operator : Logic  Operator=NOT  AllPortsSameDT=off  OutDataTypeStr=boolean
  Relational Operator : RelationalOperator  Operator=<=  OutDataTypeStr=boolean
  Timer : hcu_lib/Timer  SystemSampleTime=-1
  Valid_out : Outport
  wires:
  TimeOut/1 -> Relational Operator/2
  Relational Operator/1 -> Valid_out/1
  Logical Operator/1 -> Timer/Enable
  Rx_status/1 -> Logical Operator/1
  Timer/1 -> Relational Operator/1

== system hcu_main_ADASwEPS/dHAL_IN/HAL_IN_CANVALID/ChaekCANValid4 ==
  Rx_status : Inport
  TimeOut : Inport  Port=2
  Logical Operator : Logic  Operator=NOT  AllPortsSameDT=off  OutDataTypeStr=boolean
  Relational Operator : RelationalOperator  Operator=<=  OutDataTypeStr=boolean
  Timer : hcu_lib/Timer  SystemSampleTime=-1
  Valid_out : Outport
  wires:
  Timer/1 -> Relational Operator/1
  Rx_status/1 -> Logical Operator/1
  Logical Operator/1 -> Timer/Enable
  Relational Operator/1 -> Valid_out/1
  TimeOut/1 -> Relational Operator/2

== system hcu_main_ADASwEPS/dHAL_IN/HAL_IN_CANVALID/ChaekCANValid5 ==
  Rx_status : Inport
  TimeOut : Inport  Port=2
  Logical Operator : Logic  Operator=NOT  AllPortsSameDT=off  OutDataTypeStr=boolean
  Relational Operator : RelationalOperator  Operator=<=  OutDataTypeStr=boolean
  Timer : hcu_lib/Timer  SystemSampleTime=-1
  Valid_out : Outport
  wires:
  TimeOut/1 -> Relational Operator/2
  Relational Operator/1 -> Valid_out/1
  Logical Operator/1 -> Timer/Enable
  Rx_status/1 -> Logical Operator/1
  Timer/1 -> Relational Operator/1

== system hcu_main_ADASwEPS/dHAL_IN/HAL_IN_CANVALID/ChaekCANValid6 ==
  Rx_status : Inport
  TimeOut : Inport  Port=2
  Logical Operator : Logic  Operator=NOT  AllPortsSameDT=off  OutDataTypeStr=boolean
  Relational Operator : RelationalOperator  Operator=<=  OutDataTypeStr=boolean
  Timer : hcu_lib/Timer  SystemSampleTime=-1
  Valid_out : Outport
  wires:
  Timer/1 -> Relational Operator/1
  Rx_status/1 -> Logical Operator/1
  Logical Operator/1 -> Timer/Enable
  Relational Operator/1 -> Valid_out/1
  TimeOut/1 -> Relational Operator/2

== system hcu_main_ADASwEPS/dHAL_IN/HAL_IN_CANVALID/ChaekCANValid7 ==
  Rx_status : Inport
  TimeOut : Inport  Port=2
  Logical Operator : Logic  Operator=NOT  AllPortsSameDT=off  OutDataTypeStr=boolean
  Relational Operator : RelationalOperator  Operator=<=  OutDataTypeStr=boolean
  Timer : hcu_lib/Timer  SystemSampleTime=-1
  Valid_out : Outport
  wires:
  TimeOut/1 -> Relational Operator/2
  Relational Operator/1 -> Valid_out/1
  Logical Operator/1 -> Timer/Enable
  Rx_status/1 -> Logical Operator/1
  Timer/1 -> Relational Operator/1

== system hcu_main_ADASwEPS/dHAL_IN/HAL_IN_CANVALID/ChaekCANValid8 ==
  Rx_status : Inport
  TimeOut : Inport  Port=2
  Logical Operator : Logic  Operator=NOT  AllPortsSameDT=off  OutDataTypeStr=boolean
  Relational Operator : RelationalOperator  Operator=<=  OutDataTypeStr=boolean
  Timer : hcu_lib/Timer  SystemSampleTime=-1
  Valid_out : Outport
  wires:
  TimeOut/1 -> Relational Operator/2
  Relational Operator/1 -> Valid_out/1
  Logical Operator/1 -> Timer/Enable
  Rx_status/1 -> Logical Operator/1
  Timer/1 -> Relational Operator/1

== system hcu_main_ADASwEPS/dHAL_IN/HAL_IN_CANVALID/ChaekCANValid9 ==
  Rx_status : Inport
  TimeOut : Inport  Port=2
  Logical Operator : Logic  Operator=NOT  AllPortsSameDT=off  OutDataTypeStr=boolean
  Relational Operator : RelationalOperator  Operator=<=  OutDataTypeStr=boolean
  Timer : hcu_lib/Timer  SystemSampleTime=-1
  Valid_out : Outport
  wires:
  Timer/1 -> Relational Operator/1
  Rx_status/1 -> Logical Operator/1
  Logical Operator/1 -> Timer/Enable
  Relational Operator/1 -> Valid_out/1
  TimeOut/1 -> Relational Operator/2

== system hcu_main_ADASwEPS/dHAL_IN/HAL_IN_CSW/BO__1040_CSW1__8_CSW ==
  CAN1_Rx : Inport
  Bus Selector : BusSelector  OutputSignals=CSW1.CSW_RFogLpSw_Sta,CSW1.CSW_DimSw_Sta
  CSW_RFogLpSw_Sta : Outport
  CSW_DimSw_Sta : Outport  Port=2
  wires:
  Bus Selector/1 -> CSW_RFogLpSw_Sta/1  "<CSW_RFogLpSw_Sta>"
  CAN1_Rx/1 -> [CAN1_Rx]
  [CAN1_Rx] -> Bus Selector/1
  Bus Selector/2 -> CSW_DimSw_Sta/1  "<CSW_DimSw_Sta>"

== system hcu_main_ADASwEPS/dHAL_IN/HAL_IN_EPB/BO__928_EPB1__8_EPB ==
  CAN1_Rx : Inport
  Bus Selector : BusSelector  OutputSignals=EPB1.PB_BrakeBinStat
  PB_BrakeBinStat : Outport
  wires:
  [CAN1_Rx] -> Bus Selector/1
  CAN1_Rx/1 -> [CAN1_Rx]
  Bus Selector/1 -> PB_BrakeBinStat/1  "<PB_BrakeBinStat>"

== system hcu_main_ADASwEPS/dHAL_IN/HAL_IN_EPM/BO__1347_LKA_Left_Lane_A__8_EPM ==
  CAN2_Rx : Inport
  Bus Selector : BusSelector  OutputSignals=LKA_Left_Lane_A.Lane_Type,LKA_Left_Lane_A.Quality,LKA_Left_Lane_A.Position,LKA_Left_Lane_A.Curvature,LKA_Left_Lane_A.Curvature_Derivative,LKA_Left_Lane_A.Width_left_marking
  VHAL_LaneTypeL_enum : Outport
  VHAL_LaneQualityL_enum : Outport  Port=2
  VHAL_LaneC0L_m : Outport  Port=3
  VHAL_LaneC2L_rat : Outport  Port=4
  VHAL_LaneC3L_rat : Outport  Port=5
  VHAL_LaneMrkWidL_m : Outport  Port=6
  wires:
  [CAN2_Rx] -> Bus Selector/1
  CAN2_Rx/1 -> [CAN2_Rx]
  Bus Selector/1 -> VHAL_LaneTypeL_enum/1  "<Lane_Type>"
  Bus Selector/2 -> VHAL_LaneQualityL_enum/1  "<Quality>"
  Bus Selector/6 -> VHAL_LaneMrkWidL_m/1  "<Width_left_marking>"
  Bus Selector/3 -> VHAL_LaneC0L_m/1  "<Position>"
  Bus Selector/4 -> VHAL_LaneC2L_rat/1  "<Curvature>"
  Bus Selector/5 -> VHAL_LaneC3L_rat/1  "<Curvature_Derivative>"

== system hcu_main_ADASwEPS/dHAL_IN/HAL_IN_EPM/BO__1347_LKA_Left_Lane_B__8_EPM ==
  CAN2_Rx : Inport
  Bus Selector : BusSelector  OutputSignals=LKA_Left_Lane_B.Heading_Angle,LKA_Left_Lane_B.View_Range_Start,LKA_Left_Lane_B.View_Range_End,LKA_Left_Lane_B.Lane_Crossing,LKA_Left_Lane_B.Lane_mark_color,LKA_Left_Lane_B.TLC
  VHAL_LaneC1L_rad : Outport
  VHAL_ViewRangeStartL_m : Outport  Port=2
  VHAL_ViewRangeEndL_m : Outport  Port=3
  VHAL_LaneCrossingL_flg : Outport  Port=4
  VHAL_LaneMrkClrL_enum : Outport  Port=5
  VHAL_TLCL_s : Outport  Port=6
  wires:
  Bus Selector/5 -> VHAL_LaneMrkClrL_enum/1  "<Lane_mark_color>"
  Bus Selector/4 -> VHAL_LaneCrossingL_flg/1  "<Lane_Crossing>"
  Bus Selector/3 -> VHAL_ViewRangeEndL_m/1  "<View_Range_End>"
  Bus Selector/6 -> VHAL_TLCL_s/1  "<TLC>"
  Bus Selector/2 -> VHAL_ViewRangeStartL_m/1  "<View_Range_Start>"
  Bus Selector/1 -> VHAL_LaneC1L_rad/1  "<Heading_Angle>"
  CAN2_Rx/1 -> [CAN2_Rx]
  [CAN2_Rx] -> Bus Selector/1

== system hcu_main_ADASwEPS/dHAL_IN/HAL_IN_EPM/BO__1347_LKA_Right_Lane_A__8_EPM ==
  CAN2_Rx : Inport
  Bus Selector : BusSelector  OutputSignals=LKA_Right_Lane_A.Lane_Type,LKA_Right_Lane_A.Quality,LKA_Right_Lane_A.Position,LKA_Right_Lane_A.Curvature,LKA_Right_Lane_A.Curvature_Derivative,LKA_Right_Lane_A.Width_right_marking
  VHAL_LaneTypeR_enum : Outport
  VHAL_LaneQualityR_enum : Outport  Port=2
  VHAL_LaneC0R_m : Outport  Port=3
  VHAL_LaneC2R_rat : Outport  Port=4
  VHAL_LaneC3R_rat : Outport  Port=5
  VHAL_LaneMrkWidR_m : Outport  Port=6
  wires:
  Bus Selector/5 -> VHAL_LaneC3R_rat/1  "<Curvature_Derivative>"
  Bus Selector/4 -> VHAL_LaneC2R_rat/1  "<Curvature>"
  Bus Selector/3 -> VHAL_LaneC0R_m/1  "<Position>"
  Bus Selector/6 -> VHAL_LaneMrkWidR_m/1  "<Width_right_marking>"
  Bus Selector/2 -> VHAL_LaneQualityR_enum/1  "<Quality>"
  Bus Selector/1 -> VHAL_LaneTypeR_enum/1  "<Lane_Type>"
  CAN2_Rx/1 -> [CAN2_Rx]
  [CAN2_Rx] -> Bus Selector/1

== system hcu_main_ADASwEPS/dHAL_IN/HAL_IN_EPM/BO__1347_LKA_Right_Lane_B__8_EPM ==
  CAN2_Rx : Inport
  Bus Selector : BusSelector  OutputSignals=LKA_Right_Lane_B.Heading_Angle,LKA_Right_Lane_B.View_Range_Start,LKA_Right_Lane_B.View_Range_End,LKA_Right_Lane_B.Lane_Crossing,LKA_Right_Lane_B.Lane_mark_color,LKA_Right_Lane_B.TLC
  VHAL_LaneC1R_rad : Outport
  VHAL_ViewRangeStartR_m : Outport  Port=2
  VHAL_ViewRangeEndR_m : Outport  Port=3
  VHAL_LaneCrossingR_flg : Outport  Port=4
  VHAL_LaneMrkClrR_enum : Outport  Port=5
  VHAL_TLCR_s : Outport  Port=6
  wires:
  [CAN2_Rx] -> Bus Selector/1
  CAN2_Rx/1 -> [CAN2_Rx]
  Bus Selector/1 -> VHAL_LaneC1R_rad/1  "<Heading_Angle>"
  Bus Selector/2 -> VHAL_ViewRangeStartR_m/1  "<View_Range_Start>"
  Bus Selector/6 -> VHAL_TLCR_s/1  "<TLC>"
  Bus Selector/3 -> VHAL_ViewRangeEndR_m/1  "<View_Range_End>"
  Bus Selector/4 -> VHAL_LaneCrossingR_flg/1  "<Lane_Crossing>"
  Bus Selector/5 -> VHAL_LaneMrkClrR_enum/1  "<Lane_mark_color>"

== system hcu_main_ADASwEPS/dHAL_IN/HAL_IN_EPM/BO__1848_ObstacleStatusA__8_EPM ==
  CAN2_Rx : Inport
  Bit1 : simulink/Logic and Bit Operations/Bitwise Operator  logicop=AND  UseBitMask=on  BitMask=bin2dec('0000000000000001')  BitMaskRealWorld=Stored Integer
  Bit10 : simulink/Logic and Bit Operations/Bitwise Operator  logicop=AND  UseBitMask=on  BitMask=bin2dec('0000001000000000')  BitMaskRealWorld=Stored Integer
  Bit11 : simulink/Logic and Bit Operations/Bitwise Operator  logicop=AND  UseBitMask=on  BitMask=bin2dec('0000010000000000')  BitMaskRealWorld=Stored Integer
  Bit12 : simulink/Logic and Bit Operations/Bitwise Operator  logicop=AND  UseBitMask=on  BitMask=bin2dec('0000100000000000')  BitMaskRealWorld=Stored Integer
  Bit13 : simulink/Logic and Bit Operations/Bitwise Operator  logicop=AND  UseBitMask=on  BitMask=bin2dec('0001000000000000')  BitMaskRealWorld=Stored Integer
  Bit2 : simulink/Logic and Bit Operations/Bitwise Operator  logicop=AND  UseBitMask=on  BitMask=bin2dec('0000000000000010')  BitMaskRealWorld=Stored Integer
  Bit3 : simulink/Logic and Bit Operations/Bitwise Operator  logicop=AND  UseBitMask=on  BitMask=bin2dec('0000000000000100')  BitMaskRealWorld=Stored Integer
  Bit4 : simulink/Logic and Bit Operations/Bitwise Operator  logicop=AND  UseBitMask=on  BitMask=bin2dec('0000000000001000')  BitMaskRealWorld=Stored Integer
  Bit5 : simulink/Logic and Bit Operations/Bitwise Operator  logicop=AND  UseBitMask=on  BitMask=bin2dec('0000000000010000')  BitMaskRealWorld=Stored Integer
  Bit6 : simulink/Logic and Bit Operations/Bitwise Operator  logicop=AND  UseBitMask=on  BitMask=bin2dec('0000000000100000')  BitMaskRealWorld=Stored Integer
  Bit7 : simulink/Logic and Bit Operations/Bitwise Operator  logicop=AND  UseBitMask=on  BitMask=bin2dec('0000000001000000')  BitMaskRealWorld=Stored Integer
  Bit8 : simulink/Logic and Bit Operations/Bitwise Operator  logicop=AND  UseBitMask=on  BitMask=bin2dec('0000000010000000')  BitMaskRealWorld=Stored Integer
  Bit9 : simulink/Logic and Bit Operations/Bitwise Operator  logicop=AND  UseBitMask=on  BitMask=bin2dec('0000000100000000')  BitMaskRealWorld=Stored Integer
  Bus Selector : BusSelector  OutputSignals=ObstacleStatusA.NumObstacles,ObstacleStatusA.Go,ObstacleStatusA.Close_Car,ObstacleStatusA.RightCloseRangeCutIn,ObstacleStatusA.LeftCloseRangeCutIn,ObstacleStatusA.Failsafe
  Data Type Conversion : DataTypeConversion  OutDataTypeStr=uint16
  Shift Arithmetic : ArithShift  BitShiftNumber=1  BitShiftDirection=Right
  Shift Arithmetic1 : ArithShift  BitShiftNumber=2  BitShiftDirection=Right
  Shift Arithmetic10 : ArithShift  BitShiftNumber=11  BitShiftDirection=Right
  Shift Arithmetic11 : ArithShift  BitShiftNumber=12  BitShiftDirection=Right
  Shift Arithmetic2 : ArithShift  BitShiftNumber=3  BitShiftDirection=Right
  Shift Arithmetic3 : ArithShift  BitShiftNumber=4  BitShiftDirection=Right
  Shift Arithmetic4 : ArithShift  BitShiftNumber=5  BitShiftDirection=Right
  Shift Arithmetic5 : ArithShift  BitShiftNumber=6  BitShiftDirection=Right
  Shift Arithmetic6 : ArithShift  BitShiftNumber=7  BitShiftDirection=Right
  Shift Arithmetic7 : ArithShift  BitShiftNumber=8  BitShiftDirection=Right
  Shift Arithmetic8 : ArithShift  BitShiftNumber=9  BitShiftDirection=Right
  Shift Arithmetic9 : ArithShift  BitShiftNumber=10  BitShiftDirection=Right
  VHAL_CamNofObjects_num : Outport
  VHAL_CamGoDecision_enum : Outport  Port=2
  VHAL_CloseCarDetected_flg : Outport  Port=3
  VHAL_RightCarCutIn_flg : Outport  Port=4
  VHAL_LeftCarCutIn_flg : Outport  Port=5
  VHAL_CamFSImpairedVD_flg : Outport  Port=6
  VHAL_CamFSLowSun_flg : Outport  Port=7
  VHAL_CamFSBlurImage_flg : Outport  Port=8
  VHAL_CamFSSmearImage_flg : Outport  Port=9
  VHAL_CamFSPartialBlockage_flg : Outport  Port=10
  VHAL_CamFSFullBlockage_flg : Outport  Port=11
  VHAL_CamFSSplashes_flg : Outport  Port=12
  VHAL_CamFSOutofCal_flg : Outport  Port=13
  VHAL_CamFSCalMisalign_flg : Outport  Port=14
  VHAL_CamFSSmearedspots_flg : Outport  Port=15
  VHAL_CamFSSpotHalosFrozen_flg : Outport  Port=16
  VHAL_CamFSFoggySpots_flg : Outport  Port=17
  VHAL_CamFSSunRay_flg : Outport  Port=18
  wires:
  Bus Selector/1 -> VHAL_CamNofObjects_num/1  "<NumObstacles>"
  CAN2_Rx/1 -> [CAN2_Rx]
  [CAN2_Rx] -> Bus Selector/1
  Bus Selector/2 -> VHAL_CamGoDecision_enum/1  "<Go>"
  Bus Selector/3 -> VHAL_CloseCarDetected_flg/1  "<Close_Car>"
  Bus Selector/4 -> VHAL_RightCarCutIn_flg/1  "<RightCloseRangeCutIn>"
  Bus Selector/5 -> VHAL_LeftCarCutIn_flg/1  "<LeftCloseRangeCutIn>"
  Bit2/1 -> Shift Arithmetic/1
  Bit3/1 -> Shift Arithmetic1/1
  Bit4/1 -> Shift Arithmetic2/1
  Bit5/1 -> Shift Arithmetic3/1
  Bit6/1 -> Shift Arithmetic4/1
  Data Type Conversion/1 -> Bit5/1, Bit6/1, Bit12/1, Bit13/1, Bit11/1, Bit10/1, Bit9/1, Bit8/1, Bit7/1, Bit4/1, Bit3/1, Bit2/1, Bit1/1
  Bit7/1 -> Shift Arithmetic5/1
  Bit8/1 -> Shift Arithmetic6/1
  Bit9/1 -> Shift Arithmetic7/1
  Bit10/1 -> Shift Arithmetic8/1
  Bit11/1 -> Shift Arithmetic9/1
  Bit12/1 -> Shift Arithmetic10/1
  Bit13/1 -> Shift Arithmetic11/1
  Bus Selector/6 -> Data Type Conversion/1  "<Failsafe>"
  Bit1/1 -> VHAL_CamFSImpairedVD_flg/1
  Shift Arithmetic/1 -> VHAL_CamFSLowSun_flg/1
  Shift Arithmetic1/1 -> VHAL_CamFSBlurImage_flg/1
  Shift Arithmetic2/1 -> VHAL_CamFSSmearImage_flg/1
  Shift Arithmetic3/1 -> VHAL_CamFSPartialBlockage_flg/1
  Shift Arithmetic4/1 -> VHAL_CamFSFullBlockage_flg/1
  Shift Arithmetic5/1 -> VHAL_CamFSSplashes_flg/1
  Shift Arithmetic6/1 -> VHAL_CamFSOutofCal_flg/1
  Shift Arithmetic7/1 -> VHAL_CamFSCalMisalign_flg/1
  Shift Arithmetic8/1 -> VHAL_CamFSSmearedspots_flg/1
  Shift Arithmetic9/1 -> VHAL_CamFSSpotHalosFrozen_flg/1
  Shift Arithmetic10/1 -> VHAL_CamFSFoggySpots_flg/1
  Shift Arithmetic11/1 -> VHAL_CamFSSunRay_flg/1
